simulink model "All_Experiments"  (R2020b)
settings: Solver=VariableStepAuto  StartTime=0.0  StopTime=0.4  RelTol=1e-3
libraries: NeuroModelerLibrary x28
settings Model: Creator=Александра  LastModifiedBy=Bakhshiev

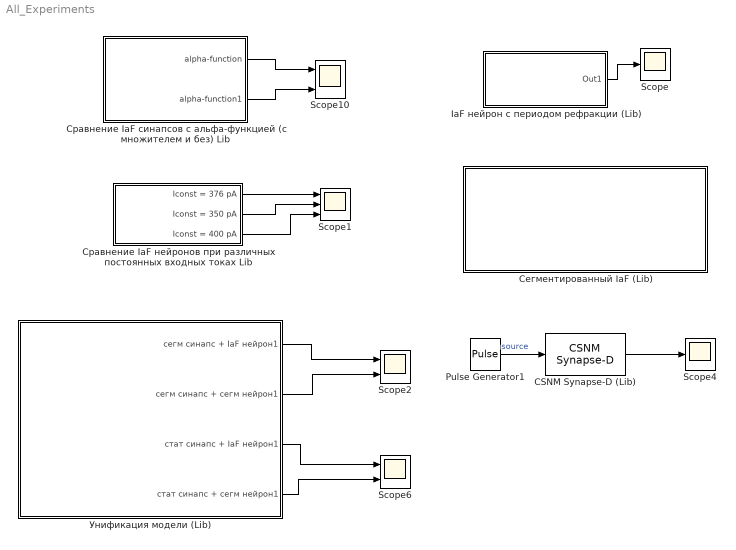
== system All_Experiments ==
  CSNM Synapse-D (Lib) : NeuroModelerLibrary/Neuron Elements/CSNM Synapse-D  SecretionTC=0.001  DecompositionTC=0.005  UseKsi=off  Rs=2e7  ksi=1  U0=-0.070  Weight=1  sign=off
  IaF нейрон с периодом рефракции (Lib) : Subsystem
  Pulse Generator1 : DiscretePulseGenerator  PulseType=Time based  Period=0.3
  Scope : Scope
  Scope1 : Scope  NumInputPorts=3
  Scope10 : Scope  NumInputPorts=2
  Scope2 : Scope  NumInputPorts=2
  Scope4 : Scope
  Scope6 : Scope  NumInputPorts=2
  Сегментированный IaF (Lib) : Subsystem
  Сравнение IaF нейронов при различных постоянных входных токах Lib : Subsystem
  Сравнение IaF синапсов с альфа-функцией (с множителем и без) Lib : Subsystem
  Унификация модели (Lib) : Subsystem
  wires:
  IaF нейрон с периодом рефракции (Lib)/1(Out1) -> Scope/1
  Сравнение IaF синапсов с альфа-функцией (с множителем и без) Lib/1(alpha-function) -> Scope10/1
  Сравнение IaF синапсов с альфа-функцией (с множителем и без) Lib/2(alpha-function1) -> Scope10/2
  Сравнение IaF нейронов при различных постоянных входных токах Lib/1(Iconst = 376 pA) -> Scope1/1
  Сравнение IaF нейронов при различных постоянных входных токах Lib/2(Iconst = 350 pA) -> Scope1/2
  Сравнение IaF нейронов при различных постоянных входных токах Lib/3(Iconst = 400 pA) -> Scope1/3
  Унификация модели (Lib)/1(сегм синапс + IaF нейрон1) -> Scope2/1
  Унификация модели (Lib)/2(сегм синапс + сегм нейрон1) -> Scope2/2
  Унификация модели (Lib)/3(стат синапс + IaF нейрон1) -> Scope6/1
  Унификация модели (Lib)/4(стат синапс + сегм нейрон1) -> Scope6/2
  Pulse Generator1/1 -> CSNM Synapse-D (Lib)/1  "source"
  CSNM Synapse-D (Lib)/1 -> Scope4/1

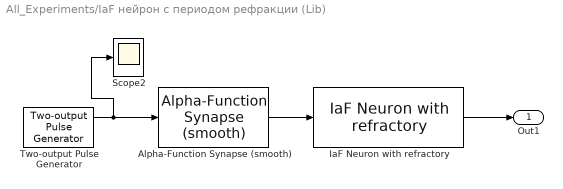
== system All_Experiments/IaF нейрон с периодом рефракции (Lib) ==
  Alpha-Function Synapse (smooth) : NeuroModelerLibrary/Classic Models/Alpha-Function Synapse (smooth)  SystemSampleTime=-1  VariantActivationTime=update diagram  Latency=0  AutoFrameSizeCalculation=off
  IaF Neuron with refractory : NeuroModelerLibrary/Classic Models/IaF Neuron with refractory  tau_m=0.01  Cm=250e-12  I_const=376e-12  E_L=-0.070  V_reset=-0.070  V_th=-0.055  tau_ref=0.002
  Scope2 : Scope
  Two-output Pulse Generator : NeuroModelerLibrary/Support/Two-output Pulse Generator  A=1  P1=200  P2=200  PW=1  ST=0.001  OOn1=0.1  OOff1=1  OOn2=1.1  OOff2=1.2
  Out1 : Outport
  wires:
  Two-output Pulse Generator/1 -> Alpha-Function Synapse (smooth)/1, Scope2/1
  Alpha-Function Synapse (smooth)/1 -> IaF Neuron with refractory/1
  IaF Neuron with refractory/1 -> Out1/1

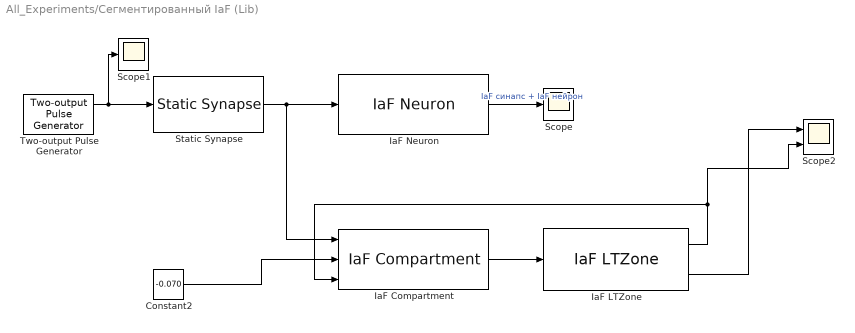
== system All_Experiments/Сегментированный IaF (Lib) ==
  Constant2 : Constant  Value=-0.070
  IaF Compartment : NeuroModelerLibrary/Neuron Elements/IaF Compartment  tau_m=0.01  Cm=250e-12  I_const=0  E_L=-0.070  V_reset=-0.10  V_th=-0.055
  IaF LTZone : NeuroModelerLibrary/Neuron Elements/IaF LTZone  tau_m=0.01  Cm=250e-12  I_const=0  E_L=-0.070  V_reset=-0.10  V_th=-0.055
  IaF Neuron : NeuroModelerLibrary/Classic Models/IaF Neuron  tau_m=0.01  Cm=250e-12  I_const=0  E_L=-0.070  V_reset=-0.10  V_th=-0.055
  Scope : Scope
  Scope1 : Scope
  Scope2 : Scope  NumInputPorts=2
  Static Synapse : NeuroModelerLibrary/Classic Models/Static Synapse  tau_syn=2e-3  I_syn=1e-8  weight=1  delay=1e-3
  Two-output Pulse Generator : NeuroModelerLibrary/Support/Two-output Pulse Generator  A=1  P1=200  P2=200  PW=1  ST=0.001  OOn1=0.1  OOff1=1  OOn2=1.1  OOff2=1.2
  wires:
  IaF LTZone/2 -> Scope2/1
  IaF LTZone/1 -> IaF Compartment/3, Scope2/2
  Constant2/1 -> IaF Compartment/2
  Two-output Pulse Generator/1 -> Static Synapse/1, Scope1/1
  IaF Neuron/1 -> Scope/1  "IaF синапс + IaF нейрон"
  Static Synapse/1 -> IaF Compartment/1, IaF Neuron/1
  IaF Compartment/1 -> IaF LTZone/1

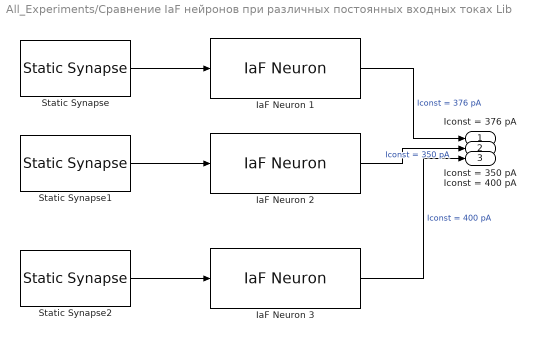
== system All_Experiments/Сравнение IaF нейронов при различных постоянных входных токах Lib ==
  IaF Neuron 1 : NeuroModelerLibrary/Classic Models/IaF Neuron  tau_m=0.01  Cm=250e-12  I_const=376e-12  E_L=-0.070  V_reset=-0.070  V_th=-0.055
  IaF Neuron 2 : NeuroModelerLibrary/Classic Models/IaF Neuron  tau_m=0.01  Cm=250e-12  I_const=350e-12  E_L=-0.070  V_reset=-0.070  V_th=-0.055
  IaF Neuron 3 : NeuroModelerLibrary/Classic Models/IaF Neuron  tau_m=0.01  Cm=250e-12  I_const=400e-12  E_L=-0.070  V_reset=-0.070  V_th=-0.055
  Static Synapse : NeuroModelerLibrary/Classic Models/Static Synapse  tau_syn=2e-3  I_syn=1e-8  weight=1  delay=1e-3
  Static Synapse1 : NeuroModelerLibrary/Classic Models/Static Synapse  tau_syn=2e-3  I_syn=1e-8  weight=1  delay=1e-3
  Static Synapse2 : NeuroModelerLibrary/Classic Models/Static Synapse  tau_syn=2e-3  I_syn=1e-8  weight=1  delay=1e-3
  Iconst = 376 pA : Outport
  Iconst = 350 pA : Outport  Port=2
  Iconst = 400 pA : Outport  Port=3
  wires:
  IaF Neuron 1/1 -> Iconst = 376 pA/1  "Iconst = 376 pA"
  Static Synapse2/1 -> IaF Neuron 3/1
  Static Synapse1/1 -> IaF Neuron 2/1
  Static Synapse/1 -> IaF Neuron 1/1
  IaF Neuron 2/1 -> Iconst = 350 pA/1  "Iconst = 350 pA"
  IaF Neuron 3/1 -> Iconst = 400 pA/1  "Iconst = 400 pA"

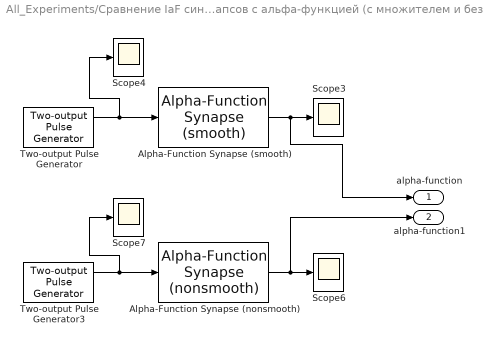
== system All_Experiments/Сравнение IaF синапсов с альфа-функцией (с множителем и без) Lib ==
  Alpha-Function Synapse (nonsmooth) : NeuroModelerLibrary/Classic Models/Alpha-Function Synapse (nonsmooth)  SystemSampleTime=-1  VariantActivationTime=update diagram  Latency=0  AutoFrameSizeCalculation=off
  Alpha-Function Synapse (smooth) : NeuroModelerLibrary/Classic Models/Alpha-Function Synapse (smooth)  SystemSampleTime=-1  VariantActivationTime=update diagram  Latency=0  AutoFrameSizeCalculation=off
  Scope{3..4,6..7} (4 alike) : Scope
  Two-output Pulse Generator : NeuroModelerLibrary/Support/Two-output Pulse Generator  A=1  P1=200  P2=200  PW=1  ST=0.001  OOn1=0.1  OOff1=1  OOn2=1.1  OOff2=1.2
  Two-output Pulse Generator3 : NeuroModelerLibrary/Support/Two-output Pulse Generator  A=1  P1=200  P2=200  PW=1  ST=0.001  OOn1=0.1  OOff1=1  OOn2=1.1  OOff2=1.2
  alpha-function : Outport
  alpha-function1 : Outport  Port=2
  wires:
  Alpha-Function Synapse (smooth)/1 -> alpha-function/1, Scope3/1
  Alpha-Function Synapse (nonsmooth)/1 -> alpha-function1/1, Scope6/1
  Two-output Pulse Generator3/1 -> Alpha-Function Synapse (nonsmooth)/1, Scope7/1
  Two-output Pulse Generator/1 -> Alpha-Function Synapse (smooth)/1, Scope4/1

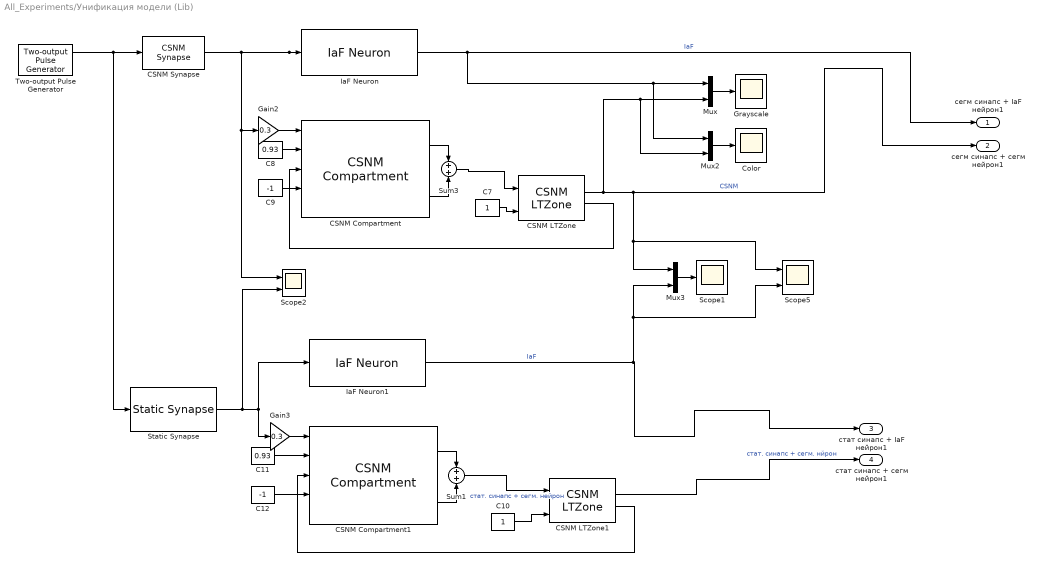
== system All_Experiments/Унификация модели (Lib) ==
  C10 : Constant
  C11 : Constant  Value=0.93
  C12 : Constant  Value=-1
  C7 : Constant
  C8 : Constant  Value=0.93
  C9 : Constant  Value=-1
  CSNM Compartment : NeuroModelerLibrary/Neuron Elements/CSNM Compartment  ACm=1e-9  ARm=1e7  ECm=1e-9  ERm=1e7  ARFm=1e7  ERFm=1e7  U0=-0.070  sign=-1
  CSNM Compartment1 : NeuroModelerLibrary/Neuron Elements/CSNM Compartment  ACm=1e-9  ARm=1e7  ECm=1e-9  ERm=1e7  ARFm=1e7  ERFm=1e7  U0=-0.070  sign=-1
  CSNM LTZone : NeuroModelerLibrary/Neuron Elements/CSNM LTZone  NM=1  FB=2  T=-0.055  switchOff=-0.1
  CSNM LTZone1 : NeuroModelerLibrary/Neuron Elements/CSNM LTZone  NM=1  FB=2  T=-0.055  switchOff=-0.1
  CSNM Synapse : NeuroModelerLibrary/Neuron Elements/CSNM Synapse  SecretionTC=0.001  DecompositionTC=0.005  UseKsi=off  Rs=2e7  ksi=1  U0=-0.070  Weight=1  sign=off
  Color : Scope
  Gain2 : Gain  Gain=0.3
  Gain3 : Gain  Gain=0.3
  Grayscale : Scope
  IaF Neuron : NeuroModelerLibrary/Classic Models/IaF Neuron  tau_m=0.01  Cm=250e-12  I_const=0  E_L=-0.070  V_reset=-0.10  V_th=-0.055
  IaF Neuron1 : NeuroModelerLibrary/Classic Models/IaF Neuron  tau_m=0.01  Cm=250e-12  I_const=0  E_L=-0.070  V_reset=-0.10  V_th=-0.055
  Mux : Mux  Inputs=2
  Mux2 : Mux  Inputs=2
  Mux3 : Mux  Inputs=2
  Scope1 : Scope
  Scope2 : Scope  NumInputPorts=2
  Scope5 : Scope  NumInputPorts=2
  Static Synapse : NeuroModelerLibrary/Classic Models/Static Synapse  tau_syn=2e-3  I_syn=1e-8  weight=1  delay=1e-3
  Sum1 : Sum  InputSameDT=on  SaturateOnIntegerOverflow=on  OutDataTypeStr=Inherit: Same as first input
  Sum3 : Sum  InputSameDT=on  SaturateOnIntegerOverflow=on  OutDataTypeStr=Inherit: Same as first input
  Two-output Pulse Generator : NeuroModelerLibrary/Support/Two-output Pulse Generator  A=1  P1=200  P2=200  PW=1  ST=0.001  OOn1=0.1  OOff1=1  OOn2=1.1  OOff2=1.2
  сегм синапс + IaF нейрон1 : Outport
  сегм синапс + сегм нейрон1 : Outport  Port=2
  стат синапс + IaF нейрон1 : Outport  Port=3
  стат синапс + сегм нейрон1 : Outport  Port=4
  wires:
  C12/1 -> CSNM Compartment1/4
  Gain3/1 -> CSNM Compartment1/1
  Mux2/1 -> Color/1
  CSNM LTZone1/3 -> CSNM Compartment1/3
  Mux3/1 -> Scope1/1
  C11/1 -> CSNM Compartment1/2
  IaF Neuron1/1 -> стат синапс + IaF нейрон1/1, Scope5/2, Mux3/2  "IaF"
  CSNM LTZone/2 -> Mux2/2, Mux/2, Scope5/1, Mux3/1, сегм синапс + сегм нейрон1/1  "CSNM"
  Sum1/1 -> CSNM LTZone1/1  "стат. синапс + сегм. нейрон"
  Mux/1 -> Grayscale/1
  C9/1 -> CSNM Compartment/4
  C8/1 -> CSNM Compartment/2
  Sum3/1 -> CSNM LTZone/1
  IaF Neuron/1 -> Mux2/1, Mux/1, сегм синапс + IaF нейрон1/1  "IaF"
  CSNM LTZone1/2 -> стат синапс + сегм нейрон1/1  "стат. синапс + сегм. нйрон"
  Static Synapse/1 -> Scope2/2, IaF Neuron1/1, Gain3/1
  CSNM Synapse/1 -> IaF Neuron/1, Scope2/1, Gain2/1
  C10/1 -> CSNM LTZone1/2
  Gain2/1 -> CSNM Compartment/1
  CSNM Compartment1/1 -> Sum1/1
  CSNM Compartment1/2 -> Sum1/2
  CSNM LTZone/3 -> CSNM Compartment/3
  Two-output Pulse Generator/1 -> Static Synapse/1, CSNM Synapse/1
  CSNM Compartment/2 -> Sum3/2
  C7/1 -> CSNM LTZone/2
  CSNM Compartment/1 -> Sum3/1
